simulink model "photorealisticSimulationEngi"  (R2022b)
settings: Solver=FixedStepAuto  StartTime=0.0  StopTime=50  RelTol=1e-3  EnableMultiTasking=on
undefined symbols (not defined in the file): initialConditions, Lidar, UAV, uavScenarioBlock
libraries: uavsimlib x5, robotcorelib x2
settings Model: DataDictionary=uavPackageDeliveryDataDict.sldd  ModifiedByFormat=The MathWorks, Inc.  Creator=The MathWorks, Inc.  LastModifiedBy=The MathWorks, Inc.
settings SolverCC: AlgebraicLoopSolver=TrustRegion  AutoInsertRateTranBlk=on  MaxZcPerStep=1
settings DataIOCC: LimitDataPoints=on  SaveOutput=off  SaveTime=off  ReturnWorkspaceOutputs=off
settings OptimizationCC: EnhancedBackFolding=on  PassReuseOutputArgsThreshold=0  ZeroExternalMemoryAtStartup=off  ZeroInternalMemoryAtStartup=off  MaxStackSize=64  OptimizeBlockOrder=speed  DifferentSizesBufferReuse=on  OptimizationCustomize=off
settings DebuggingCC: ParameterPrecisionLossMsg=none  ParameterTunabilityLossMsg=error  UnconnectedInputMsg=warning  UnconnectedOutputMsg=warning  UnconnectedLineMsg=warning  AllowSymbolicDim=off  SFUnexpectedBacktrackingDiag=warning  SFNoUnconditionalDefaultTransitionDiag=warning  SFExecutionAtInitializationDiag=none  SFMachineParentedDataDiag=warning  ArithmeticOperatorsInVariantConditions=warning
settings HardwareCC: ProdBitPerPointer=32  ProdBitPerSizeT=32  ProdBitPerPtrDiffT=32  ProdLargestAtomicFloat=None  ProdIntDivRoundTo=Undefined  ProdEndianess=Unspecified  ProdWordSize=32  ProdHWDeviceType=Generic->Unspecified (assume 32-bit Generic)
settings ModelReferenceCC: EnableRefExpFcnMdlSchedulingChecks=on  ModelReferenceNumInstancesAllowed=Single  PropagateSignalLabelsOutOfModel=off
settings SFSimCC: SimUseLocalCustomCode=off  MATLABDynamicMemAlloc=off  CustomCodeUndefinedFunction=UseInterfaceOnly  SimTargetLang=C++
settings RTWCC: GenerateReport=on  RTWUseLocalCustomCode=off  LaunchReport=on  TargetLang=C++  DLArmComputeVersion=19.05
settings CodeAppCC: ForceParamTrailComments=on  OperatorAnnotations=on
settings GRTTargetCC: TargetLangStandard=C89/C90 (ANSI)  CodeInterfacePackaging=C++ class
settings ConfigComp: CovMetricSettings=dw  CovSaveCumulativeToWorkspaceVar=on  CovSaveSingleToWorkspaceVar=on  CovExternalEMLEnable=off

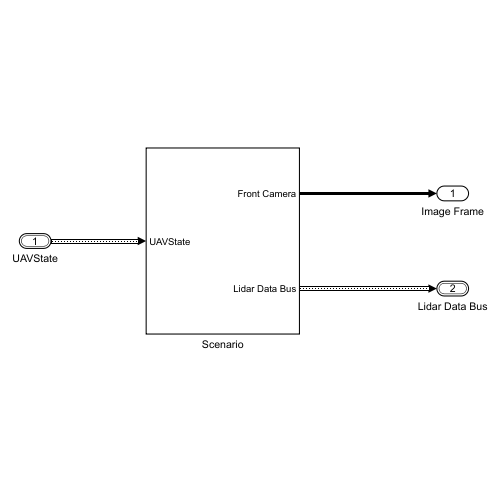
[thumbnail: Simulink's stored preview of the top-level diagram]
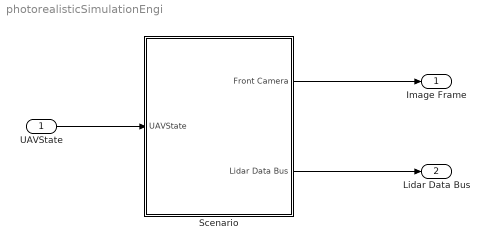
== system photorealisticSimulationEngi ==
  UAVState : Inport  OutDataTypeStr=Bus: uavStateBus  BusOutputAsStruct=on
  Scenario : Subsystem  VariantControl=isPhotoRealisticSim==1
  Image Frame : Outport
  Lidar Data Bus : Outport  Port=2  OutDataTypeStr=Bus: LidarData
  wires:
  UAVState/1 -> Scenario/1(UAVState)
  Scenario/1(Front Camera) -> Image Frame/1
  Scenario/2(Lidar Data Bus) -> Lidar Data Bus/1

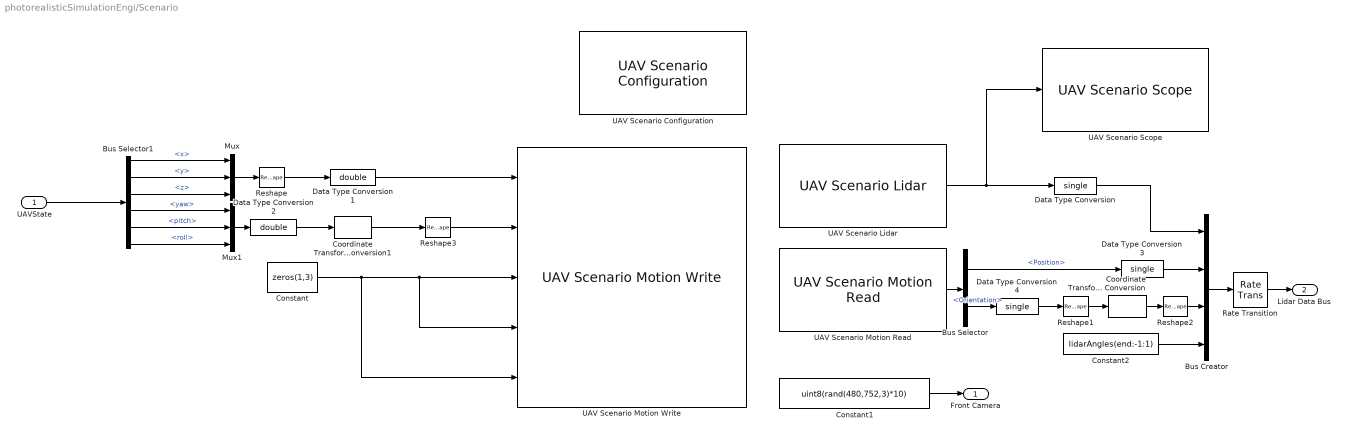
== system photorealisticSimulationEngi/Scenario ==
  UAVState : Inport
  Bus Creator : BusCreator  Inputs=4  OutDataTypeStr=Bus: LidarData  NonVirtualBus=on
      settings: InheritFromInputs=off
  Bus Selector : BusSelector  OutputSignals=Position,Orientation
  Bus Selector1 : BusSelector  OutputSignals=pos_vel.x,pos_vel.y,pos_vel.z,attitude.yaw,attitude.pitch,attitude.roll
  Constant : Constant  Value=zeros(1,3)
  Constant1 : Constant  Value=uint8(rand(480,752,3)*10)
  Constant2 : Constant  Value=lidarAngles(end:-1:1)
  Coordinate Transformation Conversion : robotcorelib/Coordinate Transformation Conversion  InputRepresentation=Quaternion  InputEulerSequence=ZYX  ShowTrVecInputPort=on  OutputRepresentation=Euler Angles  OutputEulerSequence=ZYX  ShowTrVecOutputPort=on  SimulateUsing=Code generation
  Coordinate Transformation Conversion1 : robotcorelib/Coordinate Transformation Conversion  InputRepresentation=Euler Angles  InputEulerSequence=ZYX  ShowTrVecInputPort=on  OutputRepresentation=Quaternion  OutputEulerSequence=ZYX  ShowTrVecOutputPort=on  SimulateUsing=Code generation
  Data Type Conversion : DataTypeConversion  OutDataTypeStr=single  SaturateOnIntegerOverflow=off  RndMeth=Floor
  Data Type Conversion1 : DataTypeConversion  OutDataTypeStr=double  SaturateOnIntegerOverflow=off  RndMeth=Floor
  Data Type Conversion2 : DataTypeConversion  OutDataTypeStr=double  SaturateOnIntegerOverflow=off  RndMeth=Floor
  Data Type Conversion3 : DataTypeConversion  OutDataTypeStr=single  SaturateOnIntegerOverflow=off  RndMeth=Floor
  Data Type Conversion4 : DataTypeConversion  OutDataTypeStr=single  SaturateOnIntegerOverflow=off  RndMeth=Floor
  Mux : Mux  Inputs=3
  Mux1 : Mux  Inputs=3
  Rate Transition : RateTransition  OutPortSampleTime=0.5
  Reshape : Reshape  OutputDimensionality=Row vector (2-D)
  Reshape1 : Reshape  OutputDimensionality=Column vector (2-D)
  Reshape2 : Reshape  OutputDimensionality=Row vector (2-D)
  Reshape3 : Reshape  OutputDimensionality=Row vector (2-D)
  UAV Scenario Configuration : uavsimlib/UAV Scenario Configuration  Priority=-1  UAVScenarioObject=uavScenarioBlock(initialConditions.posNED, [0 0 0])  SampleTime=0.5  UpdateParam=true  SensorMotionBusName='SensorMotionBus'  PlatformMotionBusName='PlatformMotionBus'  ScenarioMotionBusName='ScenarioMotionBus'  ScenarioMotionSignalName='ScenarioMotions'
  UAV Scenario Lidar : uavsimlib/UAV Scenario Lidar  Priority=1  SensorName=UAV/Lidar  MaxRange=90  RangeAccuracy=0.002  AzimuthLimits=[ -180, 180 ]  AzimuthResolution=0.3324099  ElevationLimits=[ -20, 20 ]  ElevationResolution=1.25  HasNoise=on  HasOrganizedOutput=on  SampleTime=0.5
  UAV Scenario Motion Read : uavsimlib/UAV Scenario Motion Read  Priority=1  EntityName='UAV/Lidar'  ReferenceFrame=NED
  UAV Scenario Motion Write : uavsimlib/UAV Scenario Motion Write  Priority=0  PlatName='UAV'  ReferenceFrame=NED
  UAV Scenario Scope : uavsimlib/UAV Scenario Scope  Priority=1  SensorNameTable={'UAV/Lidar', 'on'}  SampleTime=0.5
  Front Camera : Outport
  Lidar Data Bus : Outport  Port=2
  wires:
  Data Type Conversion2/1 -> Coordinate Transformation Conversion1/1
  Constant/1 -> UAV Scenario Motion Write/5, UAV Scenario Motion Write/4, UAV Scenario Motion Write/3
  Data Type Conversion/1 -> Bus Creator/1
  Constant1/1 -> Front Camera/1
  Bus Selector1/4 -> Mux1/1  "<yaw>"
  Mux1/1 -> Data Type Conversion2/1
  Bus Creator/1 -> Rate Transition/1
  Reshape1/1 -> Coordinate Transformation Conversion/1
  Reshape2/1 -> Bus Creator/3
  Bus Selector1/3 -> Mux/3  "<z>"
  Reshape/1 -> Data Type Conversion1/1
  Coordinate Transformation Conversion1/1 -> Reshape3/1
  Mux/1 -> Reshape/1
  Bus Selector/1 -> Data Type Conversion3/1  "<Position>"
  Reshape3/1 -> UAV Scenario Motion Write/2
  Rate Transition/1 -> Lidar Data Bus/1
  Bus Selector1/6 -> Mux1/3  "<roll>"
  Data Type Conversion4/1 -> Reshape1/1
  Data Type Conversion1/1 -> UAV Scenario Motion Write/1
  Bus Selector/2 -> Data Type Conversion4/1  "<Orientation>"
  UAV Scenario Motion Read/1 -> Bus Selector/1
  Coordinate Transformation Conversion/1 -> Reshape2/1
  Data Type Conversion3/1 -> Bus Creator/2
  UAVState/1 -> Bus Selector1/1
  Bus Selector1/5 -> Mux1/2  "<pitch>"
  Bus Selector1/2 -> Mux/2  "<y>"
  Constant2/1 -> Bus Creator/4
  UAV Scenario Lidar/1 -> UAV Scenario Scope/1, Data Type Conversion/1
  Bus Selector1/1 -> Mux/1  "<x>"
